simulink model "fmasse_var1"  (Simulink 4.00)
settings: Solver=ode45  StartTime=0.0  StopTime=10.0  RelTol=1e-3
values from neighbouring files (symbols this model uses):
  a = -1    [fmasse_var_1.m]    (also in fmasse_var_2.m; mehrw_4.m = my_system1.a; mehrw_5.m = my_system1.a)
  D1 = ((2*pi*f1)^2)*m1    (= 394784.176044)    [fmasse_var_1.m]    (also in fmasse_var_2.m)
  D2 = ((2*pi*f2)^2)*m2    (= 39478.4176044)    [fmasse_var_1.m]    (also in fmasse_var_2.m)
  m1 = 100    [fmasse_var_1.m]    (also in fmasse_var_2.m)
  m2 = 1000    [fmasse_var_1.m]    (also in fmasse_var_2.m)
  r1 = d1*2*sqrt(D1*m1)    [fmasse_var_1.m]    (also in fmasse_var_2.m)
  r2 = d2*2*sqrt(D2*m2)    [fmasse_var_1.m]
  Varianz = W/(2*d_t)/V    (= 180)    [fmasse_var_1.m]    (also in fmasse_var_2.m)
settings Model: LastModifiedBy=Administrator  BlockReductionOpt=off

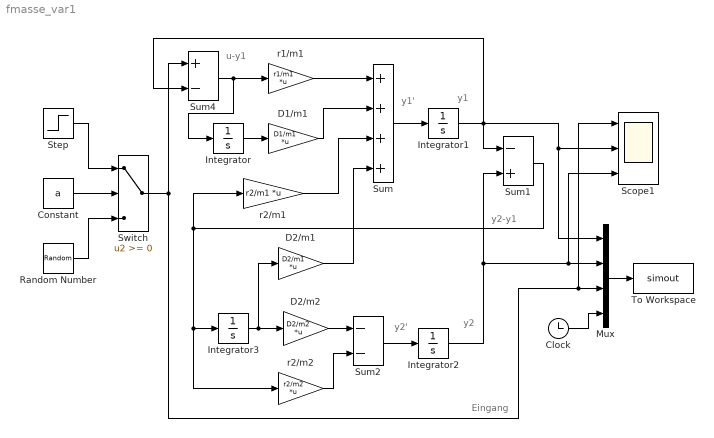
== system fmasse_var1 ==
  note: y1
  note: y1'
  note: y2
  note: y2'
  note: Eingang
  note: u-y1
  note: y2-y1
  Clock : Clock
      settings: DisplayTime=off  Decimation=10
  Constant : Constant  Value=a
  D1/m1 : Gain  Gain=D1/m1  Multiplication=Matrix(K*u)  SaturateOnIntegerOverflow=on
  D2/m1 : Gain  Gain=D2/m1  Multiplication=Matrix(K*u)  SaturateOnIntegerOverflow=on
  D2/m2 : Gain  Gain=D2/m2  Multiplication=Matrix(K*u)  SaturateOnIntegerOverflow=on
  Integrator{,1..3} (4 alike) : Integrator  ExternalReset=none  InitialConditionSource=internal  InitialCondition=0  LimitOutput=off  UpperSaturationLimit=inf  LowerSaturationLimit=-inf  ShowSaturationPort=off  ShowStatePort=off  AbsoluteTolerance=auto
  Mux : Mux  Inputs=4
  Random Number : RandomNumber  Mean=0  Variance=Varianz  Seed=0  SampleTime=0
  Scope1 : Scope  NumInputPorts=3
      settings: TimeRange=200  YMin=-15~-1~-0.8  YMax=15~0.75~0.5  SaveToWorkspace=off  MaxDataPoints=5000
  Step : Step  Time=0  Before=0  After=1  SampleTime=0
  Sum : Sum  Inputs=++++  SaturateOnIntegerOverflow=on
  Sum1 : Sum  Inputs=-+  SaturateOnIntegerOverflow=on
  Sum2 : Sum  Inputs=--  SaturateOnIntegerOverflow=on
  Sum4 : Sum  Inputs=+-  SaturateOnIntegerOverflow=on
  Switch : Switch  Threshold=0
  To Workspace : ToWorkspace  VariableName=simout  SampleTime=-1  SaveFormat=Array
  r1/m1 : Gain  Gain=r1/m1  Multiplication=Matrix(K*u)  SaturateOnIntegerOverflow=on
  r2/m1 : Gain  Gain=r2/m1  Multiplication=Matrix(K*u)  SaturateOnIntegerOverflow=on
  r2/m2 : Gain  Gain=r2/m2  Multiplication=Matrix(K*u)  SaturateOnIntegerOverflow=on
  wires:
  Mux/1 -> To Workspace/1
  Step/1 -> Switch/1
  Integrator1/1 -> Sum1/1, Sum4/2, Mux/1, Scope1/2
  Integrator2/1 -> Sum1/2, Mux/2, Scope1/3
  Sum/1 -> Integrator1/1
  r1/m1/1 -> Sum/1
  Sum4/1 -> r1/m1/1, Integrator/1
  Switch/1 -> Sum4/1, Mux/3, Scope1/1
  Integrator/1 -> D1/m1/1
  D1/m1/1 -> Sum/2
  Sum2/1 -> Integrator2/1
  D2/m2/1 -> Sum2/1
  r2/m2/1 -> Sum2/2
  r2/m1/1 -> Sum/3
  Sum1/1 -> r2/m1/1, r2/m2/1, Integrator3/1
  Integrator3/1 -> D2/m2/1, D2/m1/1
  D2/m1/1 -> Sum/4
  Clock/1 -> Mux/4
  Random Number/1 -> Switch/3
  Constant/1 -> Switch/2
